simulink model "fftanalyzeri"  (R2012b)
settings: Solver=ode3  SolverMode=SingleTasking  StartTime=0.0  StopTime=20000  RelTol=1e-3
undefined symbols (not defined in the file or in its folder): pfb_coeff_gen_calc
undefined symbols (not defined in the file): fft_bin_flags_, magphmeanmem_, threshmem_
libraries: xbsIndex_r4 x9073, casper_library_misc x119, casper_library_flow_control x51, casper_library_delays x22, xps_library x10
(part 13 of 74)

== system fftanalyzeri/FIFO64_3/FIFO32_0/FIFO16Cir_1 ==
  note: The full and empty logic is from wikipedia
      | look up FIFO on wiki.
      | No delays on emp. and full
  note: not really delayed... bad name
  note: Data valid out.
      | hith when data is good.
      | Rd is high before data is good.
  note: 6 bit addr for mem
  note: put out 8 bit addr, used for flag logic
  note: To change fifo len
      | 1. chagen me depth on dateram
      | be sure to change initial value in ram
      | 2 change ALL counter sizes
      | counters must be 1 bit more than addr width
      | 3, change all addr buss sizes
      | a pain in the ass
      | 4 change flag logic liits
  note: 2k deep
      | 36bit wide
      | 2k/16=128
      | 16 fif0s,128 len
  note: If wr addr - rdaddr <=32 then we are half full or more
  note: ram write counters
  note: write address, for full logic
      | whnen we read chan Y,
      | we want write counter for chan Y
  note: write address for chan x
  note: need z here
  note: This is a list of current addresses for each fif0, the write address.
      | Write and read act as cir buffer. tricky to tell when full..
  note: Thios is where data is stored in our multi-fifo
  note: 16 channel fifo implemented as a dual port ram
  note: Read addres counters
  note: If wr addr - rdaddr <=32 then we are half full or more
  note: If wr addr - rdaddr <=32 then we are half full or more
  chanwr : Inport
  wr : Inport  Port=2
  din : Inport  Port=3
  chanrd : Inport  Port=4
  rd : Inport  Port=5
  rst : Inport  Port=6
  rden : Inport  Port=7
  wren : Inport  Port=8
  AddSub4 : xbsIndex_r4/AddSub  mode=Subtraction  use_carryin=off  use_carryout=off  en=off  latency=0  precision=User Defined  arith_type=Unsigned  n_bits=8  bin_pt=0  quantization=Truncate  overflow=Wrap  dbl_ovrd=off  use_behavioral_HDL=off  hw_selection=Fabric  pipelined=off  block_type=addsub
  Concat : xbsIndex_r4/Concat  num_inputs=2  dbl_ovrd=off  block_type=concat
  Concat1 : xbsIndex_r4/Concat  num_inputs=2  dbl_ovrd=off  block_type=concat
  CounterArray1 : Subsystem
  CounterArray2 : Subsystem
  Inverter : xbsIndex_r4/Inverter  en=off  latency=0  dbl_ovrd=off  block_type=inv
  Inverter1 : xbsIndex_r4/Inverter  en=off  latency=0  dbl_ovrd=off  block_type=inv
  Inverter2 : xbsIndex_r4/Inverter  en=off  latency=0  dbl_ovrd=off  block_type=inv
  Logical{,1..5} (6 alike) : xbsIndex_r4/Logical  logical_function=AND  inputs=2  en=off  latency=0  precision=Full  arith_type=Unsigned  n_bits=16  bin_pt=0  align_bp=on  dbl_ovrd=off  block_type=logical
  Relational : xbsIndex_r4/Relational  mode=a=b  en=off  latency=0  dbl_ovrd=off  block_type=relational
  Relational2 : xbsIndex_r4/Relational  mode=a<=b  en=off  latency=1  dbl_ovrd=off  block_type=relational
  Relational3 : xbsIndex_r4/Relational  mode=a<=b  en=off  latency=1  dbl_ovrd=off  block_type=relational
  Relational4 : xbsIndex_r4/Relational  mode=a<=b  en=off  latency=1  dbl_ovrd=off  block_type=relational
  Relational6 : xbsIndex_r4/Relational  mode=a=b  en=off  latency=0  dbl_ovrd=off  block_type=relational
  cast_ui4_1 : xbsIndex_r4/Convert  gui_display_data_type=Fixed-point  arith_type=Unsigned  n_bits=4  bin_pt=0  float_type=Single  exp_bits=8  fraction_bits=24  quantization=Truncate  overflow=Wrap  en=off  latency=0  dbl_ovrd=off  pipeline=off  block_type=convert
  cast_ui4_2 : xbsIndex_r4/Convert  gui_display_data_type=Fixed-point  arith_type=Unsigned  n_bits=4  bin_pt=0  float_type=Single  exp_bits=8  fraction_bits=24  quantization=Truncate  overflow=Wrap  en=off  latency=0  dbl_ovrd=off  pipeline=off  block_type=convert
  dataram : xbsIndex_r4/Dual Port RAM  depth=2048  initVector=zeros(1,1024)  distributed_mem=Block RAM  init_a=0  init_b=0  rst_a=off  rst_b=off  en_a=off  en_b=off  latency=1  write_mode_A=Read Before Write  write_mode_B=Read After Write  dbl_ovrd=off  optimize=Area  use_rpm=on  block_type=dpram
  lsb7_{,1..3} (4 alike) : xbsIndex_r4/Slice  nbits=7  boolean_output=off  mode=Lower Bit Location + Width  bit1=0  base1=MSB of Input  bit0=0  base0=LSB of Input  dbl_ovrd=off  block_type=slice
  msb1_ : xbsIndex_r4/Slice  nbits=1  boolean_output=off  mode=Upper Bit Location + Width  bit1=0  base1=MSB of Input  bit0=0  base0=LSB of Input  dbl_ovrd=off  block_type=slice
  msb1_1 : xbsIndex_r4/Slice  nbits=1  boolean_output=off  mode=Upper Bit Location + Width  bit1=0  base1=MSB of Input  bit0=0  base0=LSB of Input  dbl_ovrd=off  block_type=slice
  ui6_1 : xbsIndex_r4/Constant  const=32  gui_display_data_type=Fixed-point  arith_type=Unsigned  n_bits=8  bin_pt=0  preci_type=Single  exp_width=8  frac_width=24  explicit_period=on  period=1  equ=P=C  opselect=C  inp2=PCIN>>17  opr=+  inp1=P  carry=CIN  dbl_ovrd=off  block_type=constant
  ui6_2 : xbsIndex_r4/Constant  const=16  gui_display_data_type=Fixed-point  arith_type=Unsigned  n_bits=8  bin_pt=0  preci_type=Single  exp_width=8  frac_width=24  explicit_period=on  period=1  equ=P=C  opselect=C  inp2=PCIN>>17  opr=+  inp1=P  carry=CIN  dbl_ovrd=off  block_type=constant
  ui6_3 : xbsIndex_r4/Constant  const=48  gui_display_data_type=Fixed-point  arith_type=Unsigned  n_bits=8  bin_pt=0  preci_type=Single  exp_width=8  frac_width=24  explicit_period=on  period=1  equ=P=C  opselect=C  inp2=PCIN>>17  opr=+  inp1=P  carry=CIN  dbl_ovrd=off  block_type=constant
  zero_bool_{,1..3} (4 alike) : xbsIndex_r4/Constant  const=0  gui_display_data_type=Boolean  arith_type=Boolean  n_bits=36  bin_pt=0  preci_type=Single  exp_width=8  frac_width=24  explicit_period=on  period=1  equ=P=C  opselect=C  inp2=PCIN>>17  opr=+  inp1=P  carry=CIN  dbl_ovrd=off  block_type=constant
  zero_ui36_ : xbsIndex_r4/Constant  const=0  gui_display_data_type=Fixed-point  arith_type=Unsigned  n_bits=36  bin_pt=0  preci_type=Single  exp_width=8  frac_width=24  explicit_period=on  period=1  equ=P=C  opselect=C  inp2=PCIN>>17  opr=+  inp1=P  carry=CIN  dbl_ovrd=off  block_type=constant
  q : Outport
  empty : Outport  Port=2
  halffull : Outport  Port=3
  quartfill : Outport  Port=4
  threequartfull : Outport  Port=5
  full : Outport  Port=6
  fifolen : Outport  Port=7
  dvld_out : Outport  Port=8
  wires:
  chanwr/1 -> cast_ui4_1/1
  cast_ui4_1/1 -> [channelwr]
  [channelwr] -> Concat/1
  [addr_low_wr] -> Concat/2
  Concat/1 -> [wraddr], dataram/1
  Logical1/1 -> [wr_z], dataram/3
  din/1 -> dataram/2
  Logical/1 -> [rd_z]
  cast_ui4_2/1 -> [channelrd]
  chanrd/1 -> cast_ui4_2/1
  [channelrd] -> Concat1/1
  [addr_low_rd] -> Concat1/2
  Concat1/1 -> [rdaddr], dataram/4
  zero_ui36_/1 -> dataram/5
  zero_bool_/1 -> dataram/6
  dataram/2 -> q/1
  [channelwr] -> CounterArray2/1(chan)
  CounterArray2/1(Out1) -> lsb7_/1, [addr_low_wr_b]
  [channelrd] -> CounterArray1/1(chan)
  CounterArray1/1(Out1) -> [addr_low_rd_b], lsb7_1/1
  [channelrd] -> CounterArray2/4(chan2)
  ui6_1/1 -> Relational2/1
  Relational2/1 -> halffull/1
  rst/1 -> [rst]
  [rst] -> CounterArray2/3(rst)
  [rst] -> CounterArray1/3(rst)
  rd/1 -> Logical/1
  rden/1 -> Logical/2
  wr/1 -> Logical1/1
  wren/1 -> Logical1/2
  ui6_2/1 -> Relational3/1
  Relational3/1 -> quartfill/1
  ui6_3/1 -> Relational4/1
  Relational4/1 -> threequartfull/1
  CounterArray2/2(Out2) -> [addr_low_wr_rd_b]
  lsb7_/1 -> [addr_low_wr]
  lsb7_1/1 -> [addr_low_rd]
  [addr_low_wr_rd_b] -> AddSub4/1
  AddSub4/1 -> fifolen/1, [fifo_len]
  [addr_low_rd_b] -> AddSub4/2
  [fifo_len] -> Relational2/2
  [fifo_len] -> Relational3/2
  [fifo_len] -> Relational4/2
  Logical2/1 -> CounterArray2/2(inc)
  [wr_z] -> Logical2/1
  Inverter/1 -> [nfull]
  [nfull] -> Logical2/2
  Logical3/1 -> CounterArray1/2(inc)
  [rd_z] -> Logical3/1
  Inverter1/1 -> [nempty]
  [nempty] -> Logical3/2
  [addr_low_wr_rd_b] -> msb1_/1, lsb7_2/1
  [addr_low_rd_b] -> msb1_1/1, lsb7_3/1
  lsb7_2/1 -> Relational/1
  lsb7_3/1 -> Relational/2
  msb1_/1 -> Relational6/1
  msb1_1/1 -> Relational6/2
  Relational/1 -> [cnt_eq_lsb]
  Relational6/1 -> [cnt_eq_msb]
  [cnt_eq_lsb] -> Logical4/1
  [cnt_eq_msb] -> Logical4/2
  Logical4/1 -> Inverter1/1, empty/1, [emptyy]
  [cnt_eq_lsb] -> Logical5/1
  [cnt_eq_msb] -> Inverter2/1
  Logical5/1 -> Inverter/1, full/1
  Inverter2/1 -> Logical5/2
  [rd_z] -> dvld_out/1

== system fftanalyzeri/FIFO64_3/FIFO32_0/FIFO16Cir_2 ==
  note: The full and empty logic is from wikipedia
      | look up FIFO on wiki.
      | No delays on emp. and full
  note: not really delayed... bad name
  note: Data valid out.
      | hith when data is good.
      | Rd is high before data is good.
  note: 6 bit addr for mem
  note: put out 8 bit addr, used for flag logic
  note: To change fifo len
      | 1. chagen me depth on dateram
      | be sure to change initial value in ram
      | 2 change ALL counter sizes
      | counters must be 1 bit more than addr width
      | 3, change all addr buss sizes
      | a pain in the ass
      | 4 change flag logic liits
  note: 2k deep
      | 36bit wide
      | 2k/16=128
      | 16 fif0s,128 len
  note: If wr addr - rdaddr <=32 then we are half full or more
  note: ram write counters
  note: write address, for full logic
      | whnen we read chan Y,
      | we want write counter for chan Y
  note: write address for chan x
  note: need z here
  note: This is a list of current addresses for each fif0, the write address.
      | Write and read act as cir buffer. tricky to tell when full..
  note: Thios is where data is stored in our multi-fifo
  note: 16 channel fifo implemented as a dual port ram
  note: Read addres counters
  note: If wr addr - rdaddr <=32 then we are half full or more
  note: If wr addr - rdaddr <=32 then we are half full or more
  chanwr : Inport
  wr : Inport  Port=2
  din : Inport  Port=3
  chanrd : Inport  Port=4
  rd : Inport  Port=5
  rst : Inport  Port=6
  rden : Inport  Port=7
  wren : Inport  Port=8
  AddSub4 : xbsIndex_r4/AddSub  mode=Subtraction  use_carryin=off  use_carryout=off  en=off  latency=0  precision=User Defined  arith_type=Unsigned  n_bits=8  bin_pt=0  quantization=Truncate  overflow=Wrap  dbl_ovrd=off  use_behavioral_HDL=off  hw_selection=Fabric  pipelined=off  block_type=addsub
  Concat : xbsIndex_r4/Concat  num_inputs=2  dbl_ovrd=off  block_type=concat
  Concat1 : xbsIndex_r4/Concat  num_inputs=2  dbl_ovrd=off  block_type=concat
  CounterArray1 : Subsystem
  CounterArray2 : Subsystem
  Inverter : xbsIndex_r4/Inverter  en=off  latency=0  dbl_ovrd=off  block_type=inv
  Inverter1 : xbsIndex_r4/Inverter  en=off  latency=0  dbl_ovrd=off  block_type=inv
  Inverter2 : xbsIndex_r4/Inverter  en=off  latency=0  dbl_ovrd=off  block_type=inv
  Logical{,1..5} (6 alike) : xbsIndex_r4/Logical  logical_function=AND  inputs=2  en=off  latency=0  precision=Full  arith_type=Unsigned  n_bits=16  bin_pt=0  align_bp=on  dbl_ovrd=off  block_type=logical
  Relational : xbsIndex_r4/Relational  mode=a=b  en=off  latency=0  dbl_ovrd=off  block_type=relational
  Relational2 : xbsIndex_r4/Relational  mode=a<=b  en=off  latency=1  dbl_ovrd=off  block_type=relational
  Relational3 : xbsIndex_r4/Relational  mode=a<=b  en=off  latency=1  dbl_ovrd=off  block_type=relational
  Relational4 : xbsIndex_r4/Relational  mode=a<=b  en=off  latency=1  dbl_ovrd=off  block_type=relational
  Relational6 : xbsIndex_r4/Relational  mode=a=b  en=off  latency=0  dbl_ovrd=off  block_type=relational
  cast_ui4_1 : xbsIndex_r4/Convert  gui_display_data_type=Fixed-point  arith_type=Unsigned  n_bits=4  bin_pt=0  float_type=Single  exp_bits=8  fraction_bits=24  quantization=Truncate  overflow=Wrap  en=off  latency=0  dbl_ovrd=off  pipeline=off  block_type=convert
  cast_ui4_2 : xbsIndex_r4/Convert  gui_display_data_type=Fixed-point  arith_type=Unsigned  n_bits=4  bin_pt=0  float_type=Single  exp_bits=8  fraction_bits=24  quantization=Truncate  overflow=Wrap  en=off  latency=0  dbl_ovrd=off  pipeline=off  block_type=convert
  dataram : xbsIndex_r4/Dual Port RAM  depth=2048  initVector=zeros(1,1024)  distributed_mem=Block RAM  init_a=0  init_b=0  rst_a=off  rst_b=off  en_a=off  en_b=off  latency=1  write_mode_A=Read Before Write  write_mode_B=Read After Write  dbl_ovrd=off  optimize=Area  use_rpm=on  block_type=dpram
  lsb7_{,1..3} (4 alike) : xbsIndex_r4/Slice  nbits=7  boolean_output=off  mode=Lower Bit Location + Width  bit1=0  base1=MSB of Input  bit0=0  base0=LSB of Input  dbl_ovrd=off  block_type=slice
  msb1_ : xbsIndex_r4/Slice  nbits=1  boolean_output=off  mode=Upper Bit Location + Width  bit1=0  base1=MSB of Input  bit0=0  base0=LSB of Input  dbl_ovrd=off  block_type=slice
  msb1_1 : xbsIndex_r4/Slice  nbits=1  boolean_output=off  mode=Upper Bit Location + Width  bit1=0  base1=MSB of Input  bit0=0  base0=LSB of Input  dbl_ovrd=off  block_type=slice
  ui6_1 : xbsIndex_r4/Constant  const=32  gui_display_data_type=Fixed-point  arith_type=Unsigned  n_bits=8  bin_pt=0  preci_type=Single  exp_width=8  frac_width=24  explicit_period=on  period=1  equ=P=C  opselect=C  inp2=PCIN>>17  opr=+  inp1=P  carry=CIN  dbl_ovrd=off  block_type=constant
  ui6_2 : xbsIndex_r4/Constant  const=16  gui_display_data_type=Fixed-point  arith_type=Unsigned  n_bits=8  bin_pt=0  preci_type=Single  exp_width=8  frac_width=24  explicit_period=on  period=1  equ=P=C  opselect=C  inp2=PCIN>>17  opr=+  inp1=P  carry=CIN  dbl_ovrd=off  block_type=constant
  ui6_3 : xbsIndex_r4/Constant  const=48  gui_display_data_type=Fixed-point  arith_type=Unsigned  n_bits=8  bin_pt=0  preci_type=Single  exp_width=8  frac_width=24  explicit_period=on  period=1  equ=P=C  opselect=C  inp2=PCIN>>17  opr=+  inp1=P  carry=CIN  dbl_ovrd=off  block_type=constant
  zero_bool_{,1..3} (4 alike) : xbsIndex_r4/Constant  const=0  gui_display_data_type=Boolean  arith_type=Boolean  n_bits=36  bin_pt=0  preci_type=Single  exp_width=8  frac_width=24  explicit_period=on  period=1  equ=P=C  opselect=C  inp2=PCIN>>17  opr=+  inp1=P  carry=CIN  dbl_ovrd=off  block_type=constant
  zero_ui36_ : xbsIndex_r4/Constant  const=0  gui_display_data_type=Fixed-point  arith_type=Unsigned  n_bits=36  bin_pt=0  preci_type=Single  exp_width=8  frac_width=24  explicit_period=on  period=1  equ=P=C  opselect=C  inp2=PCIN>>17  opr=+  inp1=P  carry=CIN  dbl_ovrd=off  block_type=constant
  q : Outport
  empty : Outport  Port=2
  halffull : Outport  Port=3
  quartfill : Outport  Port=4
  threequartfull : Outport  Port=5
  full : Outport  Port=6
  fifolen : Outport  Port=7
  dvld_out : Outport  Port=8
  wires:
  chanwr/1 -> cast_ui4_1/1
  cast_ui4_1/1 -> [channelwr]
  [channelwr] -> Concat/1
  [addr_low_wr] -> Concat/2
  Concat/1 -> [wraddr], dataram/1
  Logical1/1 -> [wr_z], dataram/3
  din/1 -> dataram/2
  Logical/1 -> [rd_z]
  cast_ui4_2/1 -> [channelrd]
  chanrd/1 -> cast_ui4_2/1
  [channelrd] -> Concat1/1
  [addr_low_rd] -> Concat1/2
  Concat1/1 -> [rdaddr], dataram/4
  zero_ui36_/1 -> dataram/5
  zero_bool_/1 -> dataram/6
  dataram/2 -> q/1
  [channelwr] -> CounterArray2/1(chan)
  CounterArray2/1(Out1) -> lsb7_/1, [addr_low_wr_b]
  [channelrd] -> CounterArray1/1(chan)
  CounterArray1/1(Out1) -> [addr_low_rd_b], lsb7_1/1
  [channelrd] -> CounterArray2/4(chan2)
  ui6_1/1 -> Relational2/1
  Relational2/1 -> halffull/1
  rst/1 -> [rst]
  [rst] -> CounterArray2/3(rst)
  [rst] -> CounterArray1/3(rst)
  rd/1 -> Logical/1
  rden/1 -> Logical/2
  wr/1 -> Logical1/1
  wren/1 -> Logical1/2
  ui6_2/1 -> Relational3/1
  Relational3/1 -> quartfill/1
  ui6_3/1 -> Relational4/1
  Relational4/1 -> threequartfull/1
  CounterArray2/2(Out2) -> [addr_low_wr_rd_b]
  lsb7_/1 -> [addr_low_wr]
  lsb7_1/1 -> [addr_low_rd]
  [addr_low_wr_rd_b] -> AddSub4/1
  AddSub4/1 -> fifolen/1, [fifo_len]
  [addr_low_rd_b] -> AddSub4/2
  [fifo_len] -> Relational2/2
  [fifo_len] -> Relational3/2
  [fifo_len] -> Relational4/2
  Logical2/1 -> CounterArray2/2(inc)
  [wr_z] -> Logical2/1
  Inverter/1 -> [nfull]
  [nfull] -> Logical2/2
  Logical3/1 -> CounterArray1/2(inc)
  [rd_z] -> Logical3/1
  Inverter1/1 -> [nempty]
  [nempty] -> Logical3/2
  [addr_low_wr_rd_b] -> msb1_/1, lsb7_2/1
  [addr_low_rd_b] -> msb1_1/1, lsb7_3/1
  lsb7_2/1 -> Relational/1
  lsb7_3/1 -> Relational/2
  msb1_/1 -> Relational6/1
  msb1_1/1 -> Relational6/2
  Relational/1 -> [cnt_eq_lsb]
  Relational6/1 -> [cnt_eq_msb]
  [cnt_eq_lsb] -> Logical4/1
  [cnt_eq_msb] -> Logical4/2
  Logical4/1 -> Inverter1/1, empty/1, [emptyy]
  [cnt_eq_lsb] -> Logical5/1
  [cnt_eq_msb] -> Inverter2/1
  Logical5/1 -> Inverter/1, full/1
  Inverter2/1 -> Logical5/2
  [rd_z] -> dvld_out/1

== system fftanalyzeri/FIFO64_3/FIFO32_0/Subsystem ==
  chanwr : Inport
  chanrd : Inport  Port=2
  rden : Inport  Port=3
  wren : Inport  Port=4
  Inverter : xbsIndex_r4/Inverter  en=off  latency=0  dbl_ovrd=off  block_type=inv
  Inverter1 : xbsIndex_r4/Inverter  en=off  latency=0  dbl_ovrd=off  block_type=inv
  Logical{1..4} (4 alike) : xbsIndex_r4/Logical  logical_function=AND  inputs=2  en=off  latency=0  precision=Full  arith_type=Unsigned  n_bits=16  bin_pt=0  align_bp=on  dbl_ovrd=off  block_type=logical
  lsb4_ : xbsIndex_r4/Slice  nbits=1  boolean_output=on  mode=Lower Bit Location + Width  bit1=0  base1=MSB of Input  bit0=4  base0=LSB of Input  dbl_ovrd=off  block_type=slice
  lsb4_1 : xbsIndex_r4/Slice  nbits=1  boolean_output=on  mode=Lower Bit Location + Width  bit1=0  base1=MSB of Input  bit0=4  base0=LSB of Input  dbl_ovrd=off  block_type=slice
  wrl : Outport
  rdl : Outport  Port=2
  wrh : Outport  Port=3
  rdh : Outport  Port=4
  wires:
  lsb4_/1 -> Logical2/1, Inverter/1
  lsb4_1/1 -> Logical1/1, Inverter1/1
  Inverter/1 -> Logical3/1
  Inverter1/1 -> Logical4/1
  chanrd/1 -> lsb4_1/1
  chanwr/1 -> lsb4_/1
  Logical1/1 -> rdh/1
  Logical2/1 -> wrh/1
  Logical3/1 -> wrl/1
  Logical4/1 -> rdl/1
  rden/1 -> Logical4/2, Logical1/2
  wren/1 -> Logical3/2, Logical2/2

== system fftanalyzeri/FIFO64_3/FIFO32_0/Subsystem1 ==
  In1 : Inport
  In2 : Inport  Port=2
  In3 : Inport  Port=3
  In4 : Inport  Port=4
  In5 : Inport  Port=5
  In6 : Inport  Port=6
  In7 : Inport  Port=7
  In8 : Inport  Port=8
  In9 : Inport  Port=9
  In10 : Inport  Port=10
  In11 : Inport  Port=11
  In12 : Inport  Port=12
  In13 : Inport  Port=13
  In14 : Inport  Port=14
  In15 : Inport  Port=15
  In16 : Inport  Port=16
  In17 : Inport  Port=17
  Mux{,1..7} (8 alike) : xbsIndex_r4/Mux  inputs=2  en=off  latency=0  precision=Full  arith_type=Unsigned  n_bits=16  bin_pt=14  quantization=Truncate  overflow=Wrap  dbl_ovrd=off  block_type=mux
  lsb4_ : xbsIndex_r4/Slice  nbits=1  boolean_output=on  mode=Lower Bit Location + Width  bit1=0  base1=MSB of Input  bit0=4  base0=LSB of Input  dbl_ovrd=off  block_type=slice
  Out1 : Outport
  Out2 : Outport  Port=2
  Out3 : Outport  Port=3
  Out4 : Outport  Port=4
  Out5 : Outport  Port=5
  Out6 : Outport  Port=6
  Out7 : Outport  Port=7
  Out8 : Outport  Port=8
  wires:
  In9/1 -> Mux7/2
  Mux3/1 -> Out1/1
  In11/1 -> Mux/3
  Mux7/1 -> Out8/1
  Mux1/1 -> Out4/1
  Mux5/1 -> Out5/1
  In17/1 -> Mux7/3
  Mux6/1 -> Out7/1
  In8/1 -> Mux6/2
  In10/1 -> Mux3/3
  In3/1 -> Mux4/2
  In13/1 -> Mux1/3
  In14/1 -> Mux5/3
  Mux4/1 -> Out3/1
  lsb4_/1 -> Mux7/1, Mux2/1, Mux1/1, Mux/1, Mux6/1, Mux5/1, Mux4/1, Mux3/1
  In4/1 -> lsb4_/1
  In12/1 -> Mux4/3
  In16/1 -> Mux6/3
  Mux2/1 -> Out6/1
  In15/1 -> Mux2/3
  In1/1 -> Mux3/2
  In6/1 -> Mux5/2
  In5/1 -> Mux1/2
  Mux/1 -> Out2/1
  In7/1 -> Mux2/2
  In2/1 -> Mux/2

== system fftanalyzeri/FIFO64_3/FIFO32_1/FIFO16Cir_1 ==
  note: The full and empty logic is from wikipedia
      | look up FIFO on wiki.
      | No delays on emp. and full
  note: not really delayed... bad name
  note: Data valid out.
      | hith when data is good.
      | Rd is high before data is good.
  note: 6 bit addr for mem
  note: put out 8 bit addr, used for flag logic
  note: To change fifo len
      | 1. chagen me depth on dateram
      | be sure to change initial value in ram
      | 2 change ALL counter sizes
      | counters must be 1 bit more than addr width
      | 3, change all addr buss sizes
      | a pain in the ass
      | 4 change flag logic liits
  note: 2k deep
      | 36bit wide
      | 2k/16=128
      | 16 fif0s,128 len
  note: If wr addr - rdaddr <=32 then we are half full or more
  note: ram write counters
  note: write address, for full logic
      | whnen we read chan Y,
      | we want write counter for chan Y
  note: write address for chan x
  note: need z here
  note: This is a list of current addresses for each fif0, the write address.
      | Write and read act as cir buffer. tricky to tell when full..
  note: Thios is where data is stored in our multi-fifo
  note: 16 channel fifo implemented as a dual port ram
  note: Read addres counters
  note: If wr addr - rdaddr <=32 then we are half full or more
  note: If wr addr - rdaddr <=32 then we are half full or more
  chanwr : Inport
  wr : Inport  Port=2
  din : Inport  Port=3
  chanrd : Inport  Port=4
  rd : Inport  Port=5
  rst : Inport  Port=6
  rden : Inport  Port=7
  wren : Inport  Port=8
  AddSub4 : xbsIndex_r4/AddSub  mode=Subtraction  use_carryin=off  use_carryout=off  en=off  latency=0  precision=User Defined  arith_type=Unsigned  n_bits=8  bin_pt=0  quantization=Truncate  overflow=Wrap  dbl_ovrd=off  use_behavioral_HDL=off  hw_selection=Fabric  pipelined=off  block_type=addsub
  Concat : xbsIndex_r4/Concat  num_inputs=2  dbl_ovrd=off  block_type=concat
  Concat1 : xbsIndex_r4/Concat  num_inputs=2  dbl_ovrd=off  block_type=concat
  CounterArray1 : Subsystem
  CounterArray2 : Subsystem
  Inverter : xbsIndex_r4/Inverter  en=off  latency=0  dbl_ovrd=off  block_type=inv
  Inverter1 : xbsIndex_r4/Inverter  en=off  latency=0  dbl_ovrd=off  block_type=inv
  Inverter2 : xbsIndex_r4/Inverter  en=off  latency=0  dbl_ovrd=off  block_type=inv
  Logical{,1..5} (6 alike) : xbsIndex_r4/Logical  logical_function=AND  inputs=2  en=off  latency=0  precision=Full  arith_type=Unsigned  n_bits=16  bin_pt=0  align_bp=on  dbl_ovrd=off  block_type=logical
  Relational : xbsIndex_r4/Relational  mode=a=b  en=off  latency=0  dbl_ovrd=off  block_type=relational
  Relational2 : xbsIndex_r4/Relational  mode=a<=b  en=off  latency=1  dbl_ovrd=off  block_type=relational
  Relational3 : xbsIndex_r4/Relational  mode=a<=b  en=off  latency=1  dbl_ovrd=off  block_type=relational
  Relational4 : xbsIndex_r4/Relational  mode=a<=b  en=off  latency=1  dbl_ovrd=off  block_type=relational
  Relational6 : xbsIndex_r4/Relational  mode=a=b  en=off  latency=0  dbl_ovrd=off  block_type=relational
  cast_ui4_1 : xbsIndex_r4/Convert  gui_display_data_type=Fixed-point  arith_type=Unsigned  n_bits=4  bin_pt=0  float_type=Single  exp_bits=8  fraction_bits=24  quantization=Truncate  overflow=Wrap  en=off  latency=0  dbl_ovrd=off  pipeline=off  block_type=convert
  cast_ui4_2 : xbsIndex_r4/Convert  gui_display_data_type=Fixed-point  arith_type=Unsigned  n_bits=4  bin_pt=0  float_type=Single  exp_bits=8  fraction_bits=24  quantization=Truncate  overflow=Wrap  en=off  latency=0  dbl_ovrd=off  pipeline=off  block_type=convert
  dataram : xbsIndex_r4/Dual Port RAM  depth=2048  initVector=zeros(1,1024)  distributed_mem=Block RAM  init_a=0  init_b=0  rst_a=off  rst_b=off  en_a=off  en_b=off  latency=1  write_mode_A=Read Before Write  write_mode_B=Read After Write  dbl_ovrd=off  optimize=Area  use_rpm=on  block_type=dpram
  lsb7_{,1..3} (4 alike) : xbsIndex_r4/Slice  nbits=7  boolean_output=off  mode=Lower Bit Location + Width  bit1=0  base1=MSB of Input  bit0=0  base0=LSB of Input  dbl_ovrd=off  block_type=slice
  msb1_ : xbsIndex_r4/Slice  nbits=1  boolean_output=off  mode=Upper Bit Location + Width  bit1=0  base1=MSB of Input  bit0=0  base0=LSB of Input  dbl_ovrd=off  block_type=slice
  msb1_1 : xbsIndex_r4/Slice  nbits=1  boolean_output=off  mode=Upper Bit Location + Width  bit1=0  base1=MSB of Input  bit0=0  base0=LSB of Input  dbl_ovrd=off  block_type=slice
  ui6_1 : xbsIndex_r4/Constant  const=32  gui_display_data_type=Fixed-point  arith_type=Unsigned  n_bits=8  bin_pt=0  preci_type=Single  exp_width=8  frac_width=24  explicit_period=on  period=1  equ=P=C  opselect=C  inp2=PCIN>>17  opr=+  inp1=P  carry=CIN  dbl_ovrd=off  block_type=constant
  ui6_2 : xbsIndex_r4/Constant  const=16  gui_display_data_type=Fixed-point  arith_type=Unsigned  n_bits=8  bin_pt=0  preci_type=Single  exp_width=8  frac_width=24  explicit_period=on  period=1  equ=P=C  opselect=C  inp2=PCIN>>17  opr=+  inp1=P  carry=CIN  dbl_ovrd=off  block_type=constant
  ui6_3 : xbsIndex_r4/Constant  const=48  gui_display_data_type=Fixed-point  arith_type=Unsigned  n_bits=8  bin_pt=0  preci_type=Single  exp_width=8  frac_width=24  explicit_period=on  period=1  equ=P=C  opselect=C  inp2=PCIN>>17  opr=+  inp1=P  carry=CIN  dbl_ovrd=off  block_type=constant
  zero_bool_{,1..3} (4 alike) : xbsIndex_r4/Constant  const=0  gui_display_data_type=Boolean  arith_type=Boolean  n_bits=36  bin_pt=0  preci_type=Single  exp_width=8  frac_width=24  explicit_period=on  period=1  equ=P=C  opselect=C  inp2=PCIN>>17  opr=+  inp1=P  carry=CIN  dbl_ovrd=off  block_type=constant
  zero_ui36_ : xbsIndex_r4/Constant  const=0  gui_display_data_type=Fixed-point  arith_type=Unsigned  n_bits=36  bin_pt=0  preci_type=Single  exp_width=8  frac_width=24  explicit_period=on  period=1  equ=P=C  opselect=C  inp2=PCIN>>17  opr=+  inp1=P  carry=CIN  dbl_ovrd=off  block_type=constant
  q : Outport
  empty : Outport  Port=2
  halffull : Outport  Port=3
  quartfill : Outport  Port=4
  threequartfull : Outport  Port=5
  full : Outport  Port=6
  fifolen : Outport  Port=7
  dvld_out : Outport  Port=8
  wires:
  chanwr/1 -> cast_ui4_1/1
  cast_ui4_1/1 -> [channelwr]
  [channelwr] -> Concat/1
  [addr_low_wr] -> Concat/2
  Concat/1 -> [wraddr], dataram/1
  Logical1/1 -> [wr_z], dataram/3
  din/1 -> dataram/2
  Logical/1 -> [rd_z]
  cast_ui4_2/1 -> [channelrd]
  chanrd/1 -> cast_ui4_2/1
  [channelrd] -> Concat1/1
  [addr_low_rd] -> Concat1/2
  Concat1/1 -> [rdaddr], dataram/4
  zero_ui36_/1 -> dataram/5
  zero_bool_/1 -> dataram/6
  dataram/2 -> q/1
  [channelwr] -> CounterArray2/1(chan)
  CounterArray2/1(Out1) -> lsb7_/1, [addr_low_wr_b]
  [channelrd] -> CounterArray1/1(chan)
  CounterArray1/1(Out1) -> [addr_low_rd_b], lsb7_1/1
  [channelrd] -> CounterArray2/4(chan2)
  ui6_1/1 -> Relational2/1
  Relational2/1 -> halffull/1
  rst/1 -> [rst]
  [rst] -> CounterArray2/3(rst)
  [rst] -> CounterArray1/3(rst)
  rd/1 -> Logical/1
  rden/1 -> Logical/2
  wr/1 -> Logical1/1
  wren/1 -> Logical1/2
  ui6_2/1 -> Relational3/1
  Relational3/1 -> quartfill/1
  ui6_3/1 -> Relational4/1
  Relational4/1 -> threequartfull/1
  CounterArray2/2(Out2) -> [addr_low_wr_rd_b]
  lsb7_/1 -> [addr_low_wr]
  lsb7_1/1 -> [addr_low_rd]
  [addr_low_wr_rd_b] -> AddSub4/1
  AddSub4/1 -> fifolen/1, [fifo_len]
  [addr_low_rd_b] -> AddSub4/2
  [fifo_len] -> Relational2/2
  [fifo_len] -> Relational3/2
  [fifo_len] -> Relational4/2
  Logical2/1 -> CounterArray2/2(inc)
  [wr_z] -> Logical2/1
  Inverter/1 -> [nfull]
  [nfull] -> Logical2/2
  Logical3/1 -> CounterArray1/2(inc)
  [rd_z] -> Logical3/1
  Inverter1/1 -> [nempty]
  [nempty] -> Logical3/2
  [addr_low_wr_rd_b] -> msb1_/1, lsb7_2/1
  [addr_low_rd_b] -> msb1_1/1, lsb7_3/1
  lsb7_2/1 -> Relational/1
  lsb7_3/1 -> Relational/2
  msb1_/1 -> Relational6/1
  msb1_1/1 -> Relational6/2
  Relational/1 -> [cnt_eq_lsb]
  Relational6/1 -> [cnt_eq_msb]
  [cnt_eq_lsb] -> Logical4/1
  [cnt_eq_msb] -> Logical4/2
  Logical4/1 -> Inverter1/1, empty/1, [emptyy]
  [cnt_eq_lsb] -> Logical5/1
  [cnt_eq_msb] -> Inverter2/1
  Logical5/1 -> Inverter/1, full/1
  Inverter2/1 -> Logical5/2
  [rd_z] -> dvld_out/1

== system fftanalyzeri/FIFO64_3/FIFO32_1/FIFO16Cir_2 ==
  note: The full and empty logic is from wikipedia
      | look up FIFO on wiki.
      | No delays on emp. and full
  note: not really delayed... bad name
  note: Data valid out.
      | hith when data is good.
      | Rd is high before data is good.
  note: 6 bit addr for mem
  note: put out 8 bit addr, used for flag logic
  note: To change fifo len
      | 1. chagen me depth on dateram
      | be sure to change initial value in ram
      | 2 change ALL counter sizes
      | counters must be 1 bit more than addr width
      | 3, change all addr buss sizes
      | a pain in the ass
      | 4 change flag logic liits
  note: 2k deep
      | 36bit wide
      | 2k/16=128
      | 16 fif0s,128 len
  note: If wr addr - rdaddr <=32 then we are half full or more
  note: ram write counters
  note: write address, for full logic
      | whnen we read chan Y,
      | we want write counter for chan Y
  note: write address for chan x
  note: need z here
  note: This is a list of current addresses for each fif0, the write address.
      | Write and read act as cir buffer. tricky to tell when full..
  note: Thios is where data is stored in our multi-fifo
  note: 16 channel fifo implemented as a dual port ram
  note: Read addres counters
  note: If wr addr - rdaddr <=32 then we are half full or more
  note: If wr addr - rdaddr <=32 then we are half full or more
  chanwr : Inport
  wr : Inport  Port=2
  din : Inport  Port=3
  chanrd : Inport  Port=4
  rd : Inport  Port=5
  rst : Inport  Port=6
  rden : Inport  Port=7
  wren : Inport  Port=8
  AddSub4 : xbsIndex_r4/AddSub  mode=Subtraction  use_carryin=off  use_carryout=off  en=off  latency=0  precision=User Defined  arith_type=Unsigned  n_bits=8  bin_pt=0  quantization=Truncate  overflow=Wrap  dbl_ovrd=off  use_behavioral_HDL=off  hw_selection=Fabric  pipelined=off  block_type=addsub
  Concat : xbsIndex_r4/Concat  num_inputs=2  dbl_ovrd=off  block_type=concat
  Concat1 : xbsIndex_r4/Concat  num_inputs=2  dbl_ovrd=off  block_type=concat
  CounterArray1 : Subsystem
  CounterArray2 : Subsystem
  Inverter : xbsIndex_r4/Inverter  en=off  latency=0  dbl_ovrd=off  block_type=inv
  Inverter1 : xbsIndex_r4/Inverter  en=off  latency=0  dbl_ovrd=off  block_type=inv
  Inverter2 : xbsIndex_r4/Inverter  en=off  latency=0  dbl_ovrd=off  block_type=inv
  Logical{,1..5} (6 alike) : xbsIndex_r4/Logical  logical_function=AND  inputs=2  en=off  latency=0  precision=Full  arith_type=Unsigned  n_bits=16  bin_pt=0  align_bp=on  dbl_ovrd=off  block_type=logical
  Relational : xbsIndex_r4/Relational  mode=a=b  en=off  latency=0  dbl_ovrd=off  block_type=relational
  Relational2 : xbsIndex_r4/Relational  mode=a<=b  en=off  latency=1  dbl_ovrd=off  block_type=relational
  Relational3 : xbsIndex_r4/Relational  mode=a<=b  en=off  latency=1  dbl_ovrd=off  block_type=relational
  Relational4 : xbsIndex_r4/Relational  mode=a<=b  en=off  latency=1  dbl_ovrd=off  block_type=relational
  Relational6 : xbsIndex_r4/Relational  mode=a=b  en=off  latency=0  dbl_ovrd=off  block_type=relational
  cast_ui4_1 : xbsIndex_r4/Convert  gui_display_data_type=Fixed-point  arith_type=Unsigned  n_bits=4  bin_pt=0  float_type=Single  exp_bits=8  fraction_bits=24  quantization=Truncate  overflow=Wrap  en=off  latency=0  dbl_ovrd=off  pipeline=off  block_type=convert
  cast_ui4_2 : xbsIndex_r4/Convert  gui_display_data_type=Fixed-point  arith_type=Unsigned  n_bits=4  bin_pt=0  float_type=Single  exp_bits=8  fraction_bits=24  quantization=Truncate  overflow=Wrap  en=off  latency=0  dbl_ovrd=off  pipeline=off  block_type=convert
  dataram : xbsIndex_r4/Dual Port RAM  depth=2048  initVector=zeros(1,1024)  distributed_mem=Block RAM  init_a=0  init_b=0  rst_a=off  rst_b=off  en_a=off  en_b=off  latency=1  write_mode_A=Read Before Write  write_mode_B=Read After Write  dbl_ovrd=off  optimize=Area  use_rpm=on  block_type=dpram
  lsb7_{,1..3} (4 alike) : xbsIndex_r4/Slice  nbits=7  boolean_output=off  mode=Lower Bit Location + Width  bit1=0  base1=MSB of Input  bit0=0  base0=LSB of Input  dbl_ovrd=off  block_type=slice
  msb1_ : xbsIndex_r4/Slice  nbits=1  boolean_output=off  mode=Upper Bit Location + Width  bit1=0  base1=MSB of Input  bit0=0  base0=LSB of Input  dbl_ovrd=off  block_type=slice
  msb1_1 : xbsIndex_r4/Slice  nbits=1  boolean_output=off  mode=Upper Bit Location + Width  bit1=0  base1=MSB of Input  bit0=0  base0=LSB of Input  dbl_ovrd=off  block_type=slice
  ui6_1 : xbsIndex_r4/Constant  const=32  gui_display_data_type=Fixed-point  arith_type=Unsigned  n_bits=8  bin_pt=0  preci_type=Single  exp_width=8  frac_width=24  explicit_period=on  period=1  equ=P=C  opselect=C  inp2=PCIN>>17  opr=+  inp1=P  carry=CIN  dbl_ovrd=off  block_type=constant
  ui6_2 : xbsIndex_r4/Constant  const=16  gui_display_data_type=Fixed-point  arith_type=Unsigned  n_bits=8  bin_pt=0  preci_type=Single  exp_width=8  frac_width=24  explicit_period=on  period=1  equ=P=C  opselect=C  inp2=PCIN>>17  opr=+  inp1=P  carry=CIN  dbl_ovrd=off  block_type=constant
  ui6_3 : xbsIndex_r4/Constant  const=48  gui_display_data_type=Fixed-point  arith_type=Unsigned  n_bits=8  bin_pt=0  preci_type=Single  exp_width=8  frac_width=24  explicit_period=on  period=1  equ=P=C  opselect=C  inp2=PCIN>>17  opr=+  inp1=P  carry=CIN  dbl_ovrd=off  block_type=constant
  zero_bool_{,1..3} (4 alike) : xbsIndex_r4/Constant  const=0  gui_display_data_type=Boolean  arith_type=Boolean  n_bits=36  bin_pt=0  preci_type=Single  exp_width=8  frac_width=24  explicit_period=on  period=1  equ=P=C  opselect=C  inp2=PCIN>>17  opr=+  inp1=P  carry=CIN  dbl_ovrd=off  block_type=constant
  zero_ui36_ : xbsIndex_r4/Constant  const=0  gui_display_data_type=Fixed-point  arith_type=Unsigned  n_bits=36  bin_pt=0  preci_type=Single  exp_width=8  frac_width=24  explicit_period=on  period=1  equ=P=C  opselect=C  inp2=PCIN>>17  opr=+  inp1=P  carry=CIN  dbl_ovrd=off  block_type=constant
  q : Outport
  empty : Outport  Port=2
  halffull : Outport  Port=3
  quartfill : Outport  Port=4
  threequartfull : Outport  Port=5
  full : Outport  Port=6
  fifolen : Outport  Port=7
  dvld_out : Outport  Port=8
  wires:
  chanwr/1 -> cast_ui4_1/1
  cast_ui4_1/1 -> [channelwr]
  [channelwr] -> Concat/1
  [addr_low_wr] -> Concat/2
  Concat/1 -> [wraddr], dataram/1
  Logical1/1 -> [wr_z], dataram/3
  din/1 -> dataram/2
  Logical/1 -> [rd_z]
  cast_ui4_2/1 -> [channelrd]
  chanrd/1 -> cast_ui4_2/1
  [channelrd] -> Concat1/1
  [addr_low_rd] -> Concat1/2
  Concat1/1 -> [rdaddr], dataram/4
  zero_ui36_/1 -> dataram/5
  zero_bool_/1 -> dataram/6
  dataram/2 -> q/1
  [channelwr] -> CounterArray2/1(chan)
  CounterArray2/1(Out1) -> lsb7_/1, [addr_low_wr_b]
  [channelrd] -> CounterArray1/1(chan)
  CounterArray1/1(Out1) -> [addr_low_rd_b], lsb7_1/1
  [channelrd] -> CounterArray2/4(chan2)
  ui6_1/1 -> Relational2/1
  Relational2/1 -> halffull/1
  rst/1 -> [rst]
  [rst] -> CounterArray2/3(rst)
  [rst] -> CounterArray1/3(rst)
  rd/1 -> Logical/1
  rden/1 -> Logical/2
  wr/1 -> Logical1/1
  wren/1 -> Logical1/2
  ui6_2/1 -> Relational3/1
  Relational3/1 -> quartfill/1
  ui6_3/1 -> Relational4/1
  Relational4/1 -> threequartfull/1
  CounterArray2/2(Out2) -> [addr_low_wr_rd_b]
  lsb7_/1 -> [addr_low_wr]
  lsb7_1/1 -> [addr_low_rd]
  [addr_low_wr_rd_b] -> AddSub4/1
  AddSub4/1 -> fifolen/1, [fifo_len]
  [addr_low_rd_b] -> AddSub4/2
  [fifo_len] -> Relational2/2
  [fifo_len] -> Relational3/2
  [fifo_len] -> Relational4/2
  Logical2/1 -> CounterArray2/2(inc)
  [wr_z] -> Logical2/1
  Inverter/1 -> [nfull]
  [nfull] -> Logical2/2
  Logical3/1 -> CounterArray1/2(inc)
  [rd_z] -> Logical3/1
  Inverter1/1 -> [nempty]
  [nempty] -> Logical3/2
  [addr_low_wr_rd_b] -> msb1_/1, lsb7_2/1
  [addr_low_rd_b] -> msb1_1/1, lsb7_3/1
  lsb7_2/1 -> Relational/1
  lsb7_3/1 -> Relational/2
  msb1_/1 -> Relational6/1
  msb1_1/1 -> Relational6/2
  Relational/1 -> [cnt_eq_lsb]
  Relational6/1 -> [cnt_eq_msb]
  [cnt_eq_lsb] -> Logical4/1
  [cnt_eq_msb] -> Logical4/2
  Logical4/1 -> Inverter1/1, empty/1, [emptyy]
  [cnt_eq_lsb] -> Logical5/1
  [cnt_eq_msb] -> Inverter2/1
  Logical5/1 -> Inverter/1, full/1
  Inverter2/1 -> Logical5/2
  [rd_z] -> dvld_out/1

== system fftanalyzeri/FIFO64_3/FIFO32_1/Subsystem ==
  chanwr : Inport
  chanrd : Inport  Port=2
  rden : Inport  Port=3
  wren : Inport  Port=4
  Inverter : xbsIndex_r4/Inverter  en=off  latency=0  dbl_ovrd=off  block_type=inv
  Inverter1 : xbsIndex_r4/Inverter  en=off  latency=0  dbl_ovrd=off  block_type=inv
  Logical{1..4} (4 alike) : xbsIndex_r4/Logical  logical_function=AND  inputs=2  en=off  latency=0  precision=Full  arith_type=Unsigned  n_bits=16  bin_pt=0  align_bp=on  dbl_ovrd=off  block_type=logical
  lsb4_ : xbsIndex_r4/Slice  nbits=1  boolean_output=on  mode=Lower Bit Location + Width  bit1=0  base1=MSB of Input  bit0=4  base0=LSB of Input  dbl_ovrd=off  block_type=slice
  lsb4_1 : xbsIndex_r4/Slice  nbits=1  boolean_output=on  mode=Lower Bit Location + Width  bit1=0  base1=MSB of Input  bit0=4  base0=LSB of Input  dbl_ovrd=off  block_type=slice
  wrl : Outport
  rdl : Outport  Port=2
  wrh : Outport  Port=3
  rdh : Outport  Port=4
  wires:
  lsb4_/1 -> Logical2/1, Inverter/1
  lsb4_1/1 -> Logical1/1, Inverter1/1
  Inverter/1 -> Logical3/1
  Inverter1/1 -> Logical4/1
  chanrd/1 -> lsb4_1/1
  chanwr/1 -> lsb4_/1
  Logical1/1 -> rdh/1
  Logical2/1 -> wrh/1
  Logical3/1 -> wrl/1
  Logical4/1 -> rdl/1
  rden/1 -> Logical4/2, Logical1/2
  wren/1 -> Logical3/2, Logical2/2

== system fftanalyzeri/FIFO64_3/FIFO32_1/Subsystem1 ==
  In1 : Inport
  In2 : Inport  Port=2
  In3 : Inport  Port=3
  In4 : Inport  Port=4
  In5 : Inport  Port=5
  In6 : Inport  Port=6
  In7 : Inport  Port=7
  In8 : Inport  Port=8
  In9 : Inport  Port=9
  In10 : Inport  Port=10
  In11 : Inport  Port=11
  In12 : Inport  Port=12
  In13 : Inport  Port=13
  In14 : Inport  Port=14
  In15 : Inport  Port=15
  In16 : Inport  Port=16
  In17 : Inport  Port=17
  Mux{,1..7} (8 alike) : xbsIndex_r4/Mux  inputs=2  en=off  latency=0  precision=Full  arith_type=Unsigned  n_bits=16  bin_pt=14  quantization=Truncate  overflow=Wrap  dbl_ovrd=off  block_type=mux
  lsb4_ : xbsIndex_r4/Slice  nbits=1  boolean_output=on  mode=Lower Bit Location + Width  bit1=0  base1=MSB of Input  bit0=4  base0=LSB of Input  dbl_ovrd=off  block_type=slice
  Out1 : Outport
  Out2 : Outport  Port=2
  Out3 : Outport  Port=3
  Out4 : Outport  Port=4
  Out5 : Outport  Port=5
  Out6 : Outport  Port=6
  Out7 : Outport  Port=7
  Out8 : Outport  Port=8
  wires:
  In9/1 -> Mux7/2
  Mux3/1 -> Out1/1
  In11/1 -> Mux/3
  Mux7/1 -> Out8/1
  Mux1/1 -> Out4/1
  Mux5/1 -> Out5/1
  In17/1 -> Mux7/3
  Mux6/1 -> Out7/1
  In8/1 -> Mux6/2
  In10/1 -> Mux3/3
  In3/1 -> Mux4/2
  In13/1 -> Mux1/3
  In14/1 -> Mux5/3
  Mux4/1 -> Out3/1
  lsb4_/1 -> Mux7/1, Mux2/1, Mux1/1, Mux/1, Mux6/1, Mux5/1, Mux4/1, Mux3/1
  In4/1 -> lsb4_/1
  In12/1 -> Mux4/3
  In16/1 -> Mux6/3
  Mux2/1 -> Out6/1
  In15/1 -> Mux2/3
  In1/1 -> Mux3/2
  In6/1 -> Mux5/2
  In5/1 -> Mux1/2
  Mux/1 -> Out2/1
  In7/1 -> Mux2/2
  In2/1 -> Mux/2

== system fftanalyzeri/MemRecordPolar/Shared BRAM/calc_add ==
  note: Use behavioural HDL
      | so that gets optimised
      | to minimum logic
  note: If reading/writing words
      | smaller than 32 bits,
      | change address so
      | that addressing is
      | big endian instead of
      | little, otherwise
      | pass through
  in : Inport
  add_sub : xbsIndex_r4/AddSub  mode=Subtraction  use_carryin=off  use_carryout=off  en=off  latency=0  precision=User Defined  arith_type=Unsigned  n_bits=max(1, log2(32/data_width))  bin_pt=0  quantization=Truncate  overflow=Wrap  dbl_ovrd=off  use_behavioral_HDL=on  hw_selection=Fabric  pipelined=off  block_type=addsub
  concat : xbsIndex_r4/Concat  num_inputs=2  dbl_ovrd=off  block_type=concat
  const : xbsIndex_r4/Constant  const=max(0, 32/data_width-1)  gui_display_data_type=Fixed-point  arith_type=Unsigned  n_bits=max(1, log2(32/data_width))  bin_pt=0  preci_type=Single  exp_width=8  frac_width=24  explicit_period=on  period=sample_rate  equ=P=C  opselect=C  inp2=PCIN>>17  opr=+  inp1=P  carry=CIN  dbl_ovrd=off  block_type=constant
      settings: block_version=11.4
  convert_addr : xbsIndex_r4/Convert  gui_display_data_type=Fixed-point  arith_type=Unsigned  n_bits=addr_width  bin_pt=0  float_type=Single  exp_bits=8  fraction_bits=24  quantization=Truncate  overflow=Wrap  en=off  latency=0  dbl_ovrd=off  pipeline=off  block_type=convert
      settings: xl_area=[0, 0, 0, 0, 0, 0, 0]
  lsw : xbsIndex_r4/Slice  nbits=max(1, log2(32/data_width))  boolean_output=off  mode=Lower Bit Location + Width  bit1=0  base1=MSB of Input  bit0=0  base0=LSB of Input  dbl_ovrd=off  block_type=slice
  manipulate : xbsIndex_r4/Constant  const=min(1, floor(32/data_width) - 1)  gui_display_data_type=Fixed-point  arith_type=Unsigned  n_bits=1  bin_pt=0  preci_type=Single  exp_width=8  frac_width=24  explicit_period=on  period=sample_rate  equ=P=C  opselect=C  inp2=PCIN>>17  opr=+  inp1=P  carry=CIN  dbl_ovrd=off  block_type=constant
      settings: block_version=11.4
  msw : xbsIndex_r4/Slice  nbits=addr_width - max(1, log2(32/data_width))  boolean_output=off  mode=Upper Bit Location + Width  bit1=0  base1=MSB of Input  bit0=0  base0=LSB of Input  dbl_ovrd=off  block_type=slice
  mux : xbsIndex_r4/Mux  inputs=2  en=off  latency=0  precision=Full  arith_type=Unsigned  n_bits=16  bin_pt=14  quantization=Truncate  overflow=Wrap  dbl_ovrd=off  block_type=mux
      settings: block_version=11.4
  out : Outport
  wires:
  convert_addr/1 -> mux/2, msw/1, lsw/1
  const/1 -> add_sub/1
  lsw/1 -> add_sub/2
  mux/1 -> out/1
  manipulate/1 -> mux/1
  concat/1 -> mux/3
  msw/1 -> concat/1
  add_sub/1 -> concat/2
  in/1 -> convert_addr/1

== system fftanalyzeri/MemRecordPolar/Shared BRAM/mem ==
  note: Undo data manipulation on way in and redo on way out for simulated data
  note: Undo address
      | manipulation for
      | simulated data
  In1 : Inport
  In2 : Inport  Port=2
  In3 : Inport  Port=3
  Disregard Subsystem : xbsIndex_r4/Disregard Subsystem  Tag=discardX  block_type=disregard
  calc_add : Subsystem  mask{data_width=32, addr_width=15, sample_rate=sample_rate}
      mask prompts: data_width "data width"; addr_width "address width"; sample_rate "sample rate"
  ram : xbsIndex_r4/Single Port RAM  depth=2^addr_width  initVector=init_vals  distributed_mem=Block RAM  write_mode=Read After Write  rst=off  init_reg=0  en=off  latency=1  dbl_ovrd=off  optimize=Area  use_rpm=on  block_type=spram
  sim_addr : xbsIndex_r4/Gateway In  gui_display_data_type=Fixed-point  arith_type=Unsigned  n_bits=addr_width  bin_pt=0  preci_type=Single  exp_width=8  frac_width=24  quantization=Truncate  overflow=Wrap  period=sample_rate  dbl_ovrd=off  timing_constraint=None  locs_specified=off  LOCs={}  UseAsADC=off  ADCChannel='1'  inherit_from_input=off  hdl_port=on  block_type=gatewayin
      settings: infoedit="Gateway in block.  Converts inputs of type Simulink integer, double and fixed point to  Xilinx fixed point type.<br><br>Hardware notes:  In hardware these blocks become top level input ports."  xl_area=[0, 0, 0, 0, 0, 0, 0]  sginterface={'Nallatech'=>{'xdspkit'=>{'non_memory_mapped_port'=>'sim_addr'}},'Xilinx'=>{'jtaghwcosim'=>{'non_memory_mapped_port'=>'sim_addr'},'xdspkit'=>{'non_memory_mapped_port'=>'sim_addr'}}}
  sim_data_in : xbsIndex_r4/Gateway In  gui_display_data_type=Fixed-point  arith_type=Unsigned  n_bits=32  bin_pt=0  preci_type=Single  exp_width=8  frac_width=24  quantization=Truncate  overflow=Wrap  period=sample_rate  dbl_ovrd=off  timing_constraint=None  locs_specified=off  LOCs={}  UseAsADC=off  ADCChannel='1'  inherit_from_input=off  hdl_port=on  block_type=gatewayin
      settings: xl_area=[0, 0, 0, 0, 0, 0, 0]  sginterface={'Nallatech'=>{'xdspkit'=>{'non_memory_mapped_port'=>'sim_data_in'}},'Xilinx'=>{'jtaghwcosim'=>{'non_memory_mapped_port'=>'sim_data_in'},'xdspkit'=>{'non_memory_mapped_port'=>'sim_data_in'}}}
  sim_data_out : xbsIndex_r4/Gateway Out  inherit_from_input=off  hdl_port=on  timing_constraint=None  locs_specified=off  LOCs={'B21','B22','A22','B23','B19','C19','A20','A21','A23','B24','A24','A25','E18','D18','C18','B18'}  UseAsDAC=off  DACChannel='1'  block_type=gatewayout
      settings: infoedit="Gateway out block.  Converts Xilinx fixed point inputs into ouputs of type Simulink integer, double, or fixed point.<P><P>Hardware notes:  In hardware these blocks become top level output ports or are discarded, depending on how they are configured."  xl_area=[0, 0, 0, 0, 0, 0, 0]  sginterface={'Nallatech'=>{'xdspkit'=>{'non_memory_mapped_port'=>'sim_data_out'}},'Xilinx'=>{'jtaghwcosim'=>{'non_memory_mapped_port'=>'sim_data_out'},'xdspkit'=>{'non_memory_mapped_port'=>'sim_data_out'}}}
  sim_munge_in : Subsystem  AncestorBlock=casper_library_flow_control/munge  mask(munge){divisions=1, div_size=32, order=[0], arith_type_out=Unsigned, bin_pt_out=0}
      mask prompts: divisions "Number of divisions"; div_size "Division size (bits)"; order "Division packing order"; arith_type_out "Output arithmetic type"; bin_pt_out "Output binary point"
      mask help: Splits an input bus into the specified number of divisions and then recombines them in the order specified (most significant division = 0,least = number divisions-1)
      mask init:
      | munge_init(gcb, ...
      |     'divisions', divisions, ...
      |     'div_size', div_size, ...
      |     'order', order, ...
      |     'arith_type_out', arith_type_out, ...
      |     'bin_pt_out', bin_pt_out);
      settings: AttributesFormatString=|
      | split:32
      | join:0
      | Unsigned [32,0]
      mask TypeOptions arith_type_out: Unsigned | Signed  (2's comp) | Floating-point
  sim_munge_out : Subsystem  AncestorBlock=casper_library_flow_control/munge  mask(munge){divisions=1, div_size=32, order=[0], arith_type_out=Unsigned, bin_pt_out=0}
      mask prompts: divisions "Number of divisions"; div_size "Division size (bits)"; order "Division packing order"; arith_type_out "Output arithmetic type"; bin_pt_out "Output binary point"
      mask help: Splits an input bus into the specified number of divisions and then recombines them in the order specified (most significant division = 0,least = number divisions-1)
      mask init:
      | munge_init(gcb, ...
      |     'divisions', divisions, ...
      |     'div_size', div_size, ...
      |     'order', order, ...
      |     'arith_type_out', arith_type_out, ...
      |     'bin_pt_out', bin_pt_out);
      settings: AttributesFormatString=|
      | split:32
      | join:0
      | Unsigned [32,0]
      mask TypeOptions arith_type_out: Unsigned | Signed  (2's comp) | Floating-point
  sim_we : xbsIndex_r4/Gateway In  gui_display_data_type=Fixed-point  arith_type=Boolean  n_bits=1  bin_pt=0  preci_type=Single  exp_width=8  frac_width=24  quantization=Truncate  overflow=Wrap  period=sample_rate  dbl_ovrd=off  timing_constraint=None  locs_specified=off  LOCs={}  UseAsADC=off  ADCChannel='1'  inherit_from_input=off  hdl_port=on  block_type=gatewayin
      settings: infoedit="Gateway in block.  Converts inputs of type Simulink integer, double and fixed point to  Xilinx fixed point type.<br><br>Hardware notes:  In hardware these blocks become top level input ports."  xl_area=[0, 0, 0, 0, 0, 0, 0]  sginterface={'Nallatech'=>{'xdspkit'=>{'non_memory_mapped_port'=>'sim_we'}},'Xilinx'=>{'jtaghwcosim'=>{'non_memory_mapped_port'=>'sim_we'},'xdspkit'=>{'non_memory_mapped_port'=>'sim_we'}}}
  Out1 : Outport
  wires:
  calc_add/1(out) -> ram/1
  sim_munge_out/1(dout) -> sim_data_out/1
  In1/1 -> sim_addr/1
  In2/1 -> sim_data_in/1
  sim_data_out/1 -> Out1/1
  In3/1 -> sim_we/1
  sim_addr/1 -> calc_add/1(in)
  sim_data_in/1 -> sim_munge_in/1(din)
  sim_we/1 -> ram/3
  ram/1 -> sim_munge_out/1(din)
  sim_munge_in/1(dout) -> ram/2

== system fftanalyzeri/MemRecordPolar/Shared BRAM/munge_in ==
  din : Inport
  reinterpret_out : xbsIndex_r4/Reinterpret  force_arith_type=on  arith_type=Unsigned  force_bin_pt=on  bin_pt=0  block_type=reinterpret
  dout : Outport
  wires:
  reinterpret_out/1 -> dout/1
  din/1 -> reinterpret_out/1

== system fftanalyzeri/MemRecordPolar/Shared BRAM/munge_out ==
  din : Inport
  reinterpret_out : xbsIndex_r4/Reinterpret  force_arith_type=on  arith_type=Unsigned  force_bin_pt=on  bin_pt=0  block_type=reinterpret
  dout : Outport
  wires:
  reinterpret_out/1 -> dout/1
  din/1 -> reinterpret_out/1
